simulink model "ElectricalElements"  (R2018b)
settings: Solver=ode45  StartTime=0.0  StopTime=10.0  RelTol=1e-3  EnableMultiTasking=on
settings Model: Creator=sz609516  LastModifiedBy=fhu-eba
settings DataIOCC: LimitDataPoints=on  SaveFormat=Array
settings OptimizationCC: LifeSpan=inf
settings DebuggingCC: UnderspecifiedInitializationDetection=Classic  MergeDetectMultiDrivingBlocksExec=none  SolverPrmCheckMsg=warning  StateNameClashWarn=warning  SFUnexpectedBacktrackingDiag=warning  SFNoUnconditionalDefaultTransitionDiag=warning
settings HardwareCC: ProdBitPerPointer=32  ProdBitPerSizeT=32  ProdBitPerPtrDiffT=32  ProdLargestAtomicFloat=None  ProdIntDivRoundTo=Undefined  ProdEndianess=Unspecified  ProdWordSize=32  ProdHWDeviceType=32-bit Generic
settings ModelReferenceCC: PropagateSignalLabelsOutOfModel=off
settings SFSimCC: SimUseLocalCustomCode=off
settings RTWCC: RTWUseLocalCustomCode=off
settings CodeAppCC: StateflowObjectComments=on
settings GRTTargetCC: TargetLangStandard=C89/C90 (ANSI)  GeneratePreprocessorConditionals=Disable all
settings ConfigComp: CovMetricSettings=dw  CovHtmlReporting=on  CovSaveCumulativeToWorkspaceVar=on  CovSaveSingleToWorkspaceVar=on  CovExternalEMLEnable=off

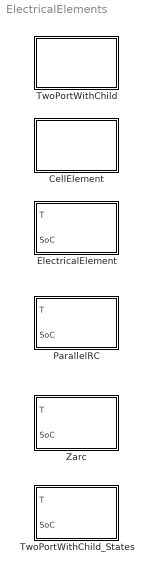
== system ElectricalElements ==
  CellElement : Subsystem
  ElectricalElement : Subsystem
  ParallelRC : Subsystem
  TwoPortWithChild : Subsystem
  TwoPortWithChild_States : Subsystem
  Zarc : Subsystem

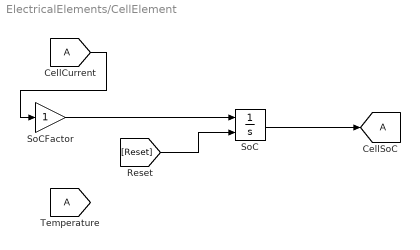
== system ElectricalElements/CellElement ==
  SoC : Integrator  ExternalReset=rising  LimitOutput=on  UpperSaturationLimit=100  LowerSaturationLimit=0
  SoCFactor : Gain
  tag scope: A=global
  wires:
  SoCFactor/1 -> SoC/1
  [A] -> SoCFactor/1
  SoC/1 -> [A]
  [Reset] -> SoC/2

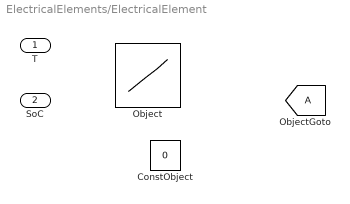
== system ElectricalElements/ElectricalElement ==
  T : Inport
  SoC : Inport  Port=2
  ConstObject : Constant  Value=0
  Object : Lookup_n-D  Table=[1,2,3;4,5,6;7,8,9]  ExtrapMethod=Clip  RndMeth=Simplest  InputSameDT=on
  tag scope: A=global

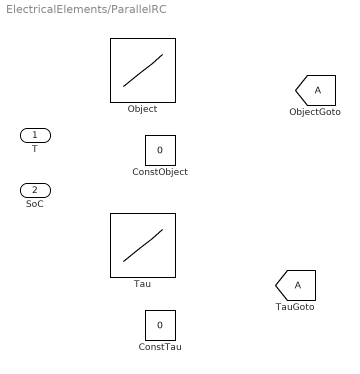
== system ElectricalElements/ParallelRC ==
  T : Inport
  SoC : Inport  Port=2
  ConstObject : Constant  Value=0
  ConstTau : Constant  Value=0
  Object : Lookup_n-D  Table=[1,2,3;4,5,6;7,8,9]  ExtrapMethod=Clip  RndMeth=Simplest  InputSameDT=on
  Tau : Lookup_n-D  Table=[1,2,3;4,5,6;7,8,9]  ExtrapMethod=Clip  RndMeth=Simplest  InputSameDT=on
  tag scope: A=global

== system ElectricalElements/TwoPortWithChild ==

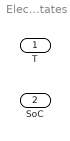
== system ElectricalElements/TwoPortWithChild_States ==
  T : Inport
  SoC : Inport  Port=2

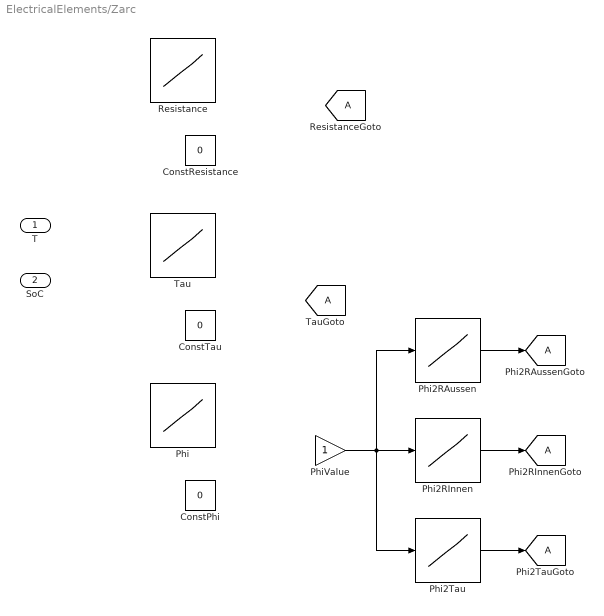
== system ElectricalElements/Zarc ==
  T : Inport
  SoC : Inport  Port=2
  ConstPhi : Constant  Value=0
  ConstResistance : Constant  Value=0
  ConstTau : Constant  Value=0
  Phi : Lookup_n-D  Table=[1,2,3;4,5,6;7,8,9]  ExtrapMethod=Clip  RndMeth=Simplest  InputSameDT=on
  Phi2RAussen : Lookup_n-D  NumberOfTableDimensions=1  BreakpointsForDimension1=[-5:5]  Table=tanh([-5:5])  ExtrapMethod=Clip  RndMeth=Simplest  InputSameDT=on
  Phi2RInnen : Lookup_n-D  NumberOfTableDimensions=1  BreakpointsForDimension1=[-5:5]  Table=tanh([-5:5])  ExtrapMethod=Clip  RndMeth=Simplest  InputSameDT=on
  Phi2Tau : Lookup_n-D  NumberOfTableDimensions=1  BreakpointsForDimension1=[-5:5]  Table=tanh([-5:5])  ExtrapMethod=Clip  RndMeth=Simplest  InputSameDT=on
  PhiValue : Gain
  Resistance : Lookup_n-D  Table=[1,2,3;4,5,6;7,8,9]  ExtrapMethod=Clip  RndMeth=Simplest  InputSameDT=on
  Tau : Lookup_n-D  Table=[1,2,3;4,5,6;7,8,9]  ExtrapMethod=Clip  RndMeth=Simplest  InputSameDT=on
  tag scope: A=global
  wires:
  Phi2RAussen/1 -> [A]
  Phi2RInnen/1 -> [A]
  Phi2Tau/1 -> [A]
  PhiValue/1 -> Phi2Tau/1, Phi2RAussen/1, Phi2RInnen/1
